simulink library "LandingGearModeLib"  (R2013b)
settings: Solver=ode45  StartTime=0.0  StopTime=10.0  RelTol=1e-3
settings Model: Creator=siddhars  LastModifiedBy=siddhars

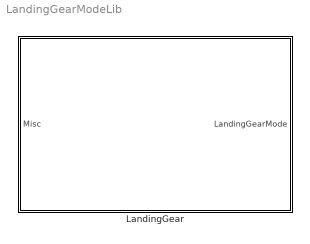
== system LandingGearModeLib ==
  LandingGear : Stateflow chart  TreatAsAtomicUnit=on

== stateflow chart LandingGearModeLib/LandingGear ==
  state LeftLock [parallel]
    settings: executionOrder=1
    state Locked
    state Unlocked
    (default) -> (junction 3)
    (junction 3) -> LeftLock.Locked [order 1] : [Misc.LGLeftLock]
    (junction 3) -> LeftLock.Unlocked [order 2]
    LeftLock.Locked -> LeftLock.Unlocked : [~Misc.LGLeftLock]
    LeftLock.Unlocked -> LeftLock.Locked : [Misc.LGLeftLock]
  state RightLock [parallel]
    settings: executionOrder=2
    state Unlocked
    state Locked
    (default) -> (junction 12)
    (junction 12) -> RightLock.Unlocked [order 2]
    (junction 12) -> RightLock.Locked [order 1] : [Misc.LGRightLock]
    RightLock.Locked -> RightLock.Unlocked : [~Misc.LGRightLock]
    RightLock.Unlocked -> RightLock.Locked : [Misc.LGRightLock]
  state WarningModes [parallel]
    settings: executionOrder=3
    state BothLocked
      entry:
      LandingGearMode = 1;
    state BothUnLocked
      entry:
      LandingGearMode = 3;
    state OnlyOneLocked
      entry:
      LandingGearMode = 2;
    state ERROR
      entry:
      LandingGearMode = 4;
    (default) -> (junction 21)
    (junction 21) -> BothLocked [order 1] : [in(LeftLock.Locked) &&...
        | in(RightLock.Locked)]
    (junction 21) -> BothUnLocked [order 2] : [in(LeftLock.Unlocked) &&...
        | in(RightLock.Unlocked)]
    (junction 21) -> OnlyOneLocked [order 3]
    BothUnLocked -> OnlyOneLocked [order 2] : [in(LeftLock.Locked) ||...
        | in(RightLock.Locked)]
    OnlyOneLocked -> BothLocked [order 3] : [in(LeftLock.Locked) &&...
        | in(RightLock.Locked)]
    OnlyOneLocked -> BothUnLocked [order 1] : [in(LeftLock.Unlocked) &&...
        | in(RightLock.Unlocked)]
    BothLocked -> OnlyOneLocked [order 2] : [in(LeftLock.Unlocked) ||...
        | in(RightLock.Unlocked)]
    OnlyOneLocked -> ERROR [order 2] : after(10,sec)
    ERROR -> OnlyOneLocked : [(in(LeftLock.Locked)&&in(RightLock.Locked)) || ...
        | (in(LeftLock.Unlocked)&&in(RightLock.Unlocked))]
    BothLocked -> BothUnLocked [order 1] : [in(LeftLock.Unlocked) &&...
        | in(RightLock.Unlocked)]
    BothUnLocked -> BothLocked [order 1] : [in(LeftLock.Locked) &&...
        | in(RightLock.Locked)]
  data: Misc input Bus: MiscData; LandingGearMode output double size=1
